simulink model "samerHARDWARE"  (R2025b)
settings: Solver=FixedStepDiscrete  StartTime=0.0  StopTime=1500  FixedStep=0.05  RelTol=1e-3
libraries: slpidlib x6
(part 1 of 2)
settings Model: SimulationMode=external  Creator=Ahmed Sedky  LastModifiedBy=Samer FARAJ
settings OptimizationCC: EnhancedBackFolding=on  PassReuseOutputArgsAs=Individual arguments  ZeroExternalMemoryAtStartup=off  ZeroInternalMemoryAtStartup=off  MaxStackSize=64  OptimizeBlockOrder=speed  DifferentSizesBufferReuse=on  OptimizationCustomize=off  EfficientTunableParamExpr=on
settings DebuggingCC: ParameterTunabilityLossMsg=error
settings HardwareCC: ProdBitPerInt=16.0  ProdBitPerPointer=16.0  ProdBitPerSizeT=16.0  ProdBitPerPtrDiffT=16.0  ProdLargestAtomicFloat=None  ProdWordSize=8.0  ProdHWDeviceType=Atmel->AVR
settings SFSimCC: MATLABDynamicMemAlloc=off
settings RTWCC: SystemTargetFile=ert.tlc  TLCOptions=-aExtModeXCPSimulationTimeInTicks=1 -aExtModeXCPClassicInterface=0  TemplateMakefile=ert_default_tmf  Toolchain=Arduino AVR  BuildConfiguration=Faster Runs  GPUComputeCapability=3.5  Description=Embedded Coder
settings CodeAppCC: ForceParamTrailComments=on  IgnoreCustomStorageClasses=off  OperatorAnnotations=on  SimulinkDataObjDesc=on  SFDataObjDesc=on  InsertBlockDesc=on
settings ERTTargetCC: ExtMode=on  ExtModeTransport=3.0  ExtModeStaticAlloc=on  ExtModeStaticAllocSize=2048.0  ExtModeMexFile=ext_xcp  ExtModeMexArgs=0 4 921600  ExtModeIntrfLevel=Level2 - Open  InlinedParameterPlacement=Hierarchical  ERTCustomFileTemplate=example_file_process.tlc  DynamicArrayContainerType=coder::array  SupportContinuousTime=on

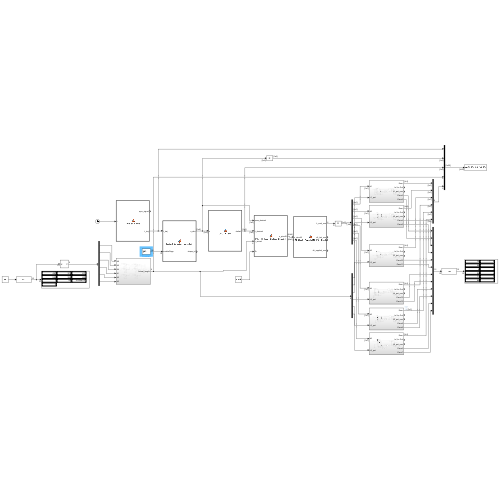
[thumbnail: Simulink's stored preview of the top-level diagram]
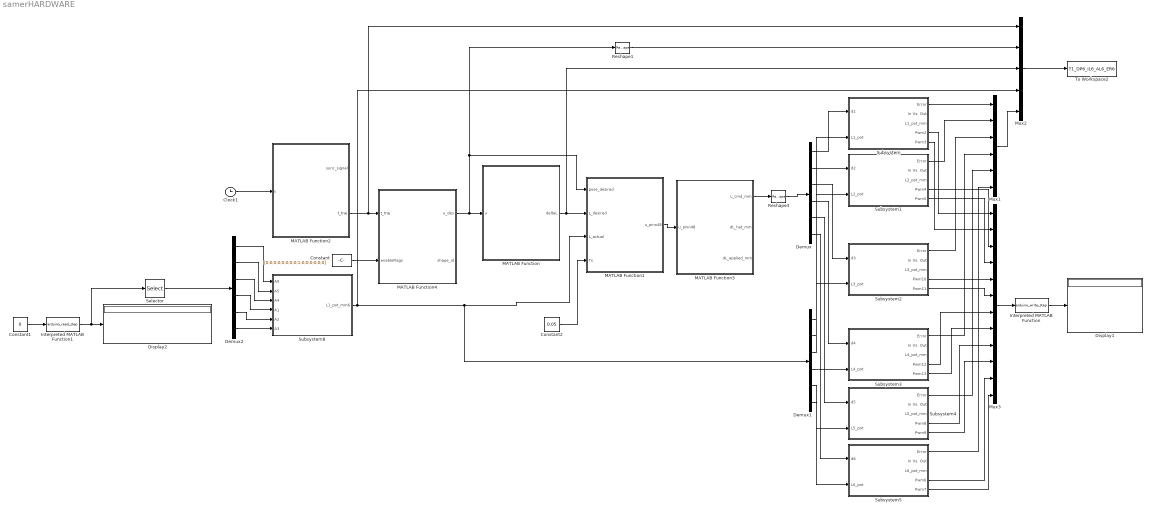
== system samerHARDWARE ==
  Clock1 : Clock
  Constant : Constant  Value=[0;0;0;0;0;0;0;0;1;0;0;0;0;0;0]
  Constant1 : Constant  Value=0
  Constant2 : Constant  Value=0.05
  Demux : Demux  Outputs=6
  Demux1 : Demux  Outputs=6
  Demux2 : Demux  Outputs=6
  Display1 : Display
  Display2 : Display
  Interpreted MATLAB Function : MATLABFcn  MATLABFcn=arduino_write_step  OutputDimensions=12  OutputSignalType=real
  Interpreted MATLAB Function1 : MATLABFcn  MATLABFcn=arduino_read_step  OutputDimensions=10  OutputSignalType=real
  MATLAB Function : MATLAB Function  TreatAsAtomicUnit=on
  MATLAB Function1 : MATLAB Function  TreatAsAtomicUnit=on
  MATLAB Function2 : MATLAB Function  TreatAsAtomicUnit=on
  MATLAB Function3 : MATLAB Function  TreatAsAtomicUnit=on
  MATLAB Function4 : MATLAB Function  TreatAsAtomicUnit=on
  Mux1 : Mux  Inputs=6
  Mux2 : Mux  Inputs=5
  Mux3 : Mux  Inputs=12
  Reshape1 : Reshape  OutputDimensionality=Customize  OutputDimensions=[1,6]
  Reshape3 : Reshape  OutputDimensionality=Customize  OutputDimensions=[1,6]
  Selector : Selector  InputPortWidth=10  IndexOptions=Index vector (dialog)  Indices=[1:6]  OutputSizes=1
  Subsystem : Subsystem
  Subsystem1 : Subsystem
  Subsystem2 : Subsystem
  Subsystem3 : Subsystem
  Subsystem4 : Subsystem
  Subsystem5 : Subsystem
  Subsystem8 : Subsystem
  To Workspace2 : ToWorkspace  VariableName=T1_DP6_IL6_AL6_ER6  SampleTime=-1
      settings: Save2DSignal=2-D array (concatenate along first dimension)
  wires:
  Constant1/1 -> Interpreted MATLAB Function1/1
  Interpreted MATLAB Function1/1 -> Selector/1, Display2/1
  Demux2/4 -> Subsystem8/4(A1)
  Demux2/3 -> Subsystem8/3(A4)
  Subsystem8/1(L1_pot_mm6) -> Demux1/1, MATLAB Function1/3(L_actual), Mux2/4
  Demux2/6 -> Subsystem8/6(A3)
  Demux2/2 -> Subsystem8/2(A5)
  Subsystem/5(Pwm3) -> Mux3/2
  Subsystem/1(Error) -> Mux1/1
  Selector/1 -> Demux2/1
  Demux1/5 -> Subsystem4/2(L5_pot)
  Demux1/1 -> Subsystem/2(L1_pot)
  Demux/5 -> Subsystem4/1(d5)
  Demux2/1 -> Subsystem8/1(A0)
  Clock1/1 -> MATLAB Function2/1(t)
  Interpreted MATLAB Function/1 -> Display1/1
  Demux2/5 -> Subsystem8/5(A2)
  Mux3/1 -> Interpreted MATLAB Function/1
  Subsystem1/1(Error) -> Mux1/2
  MATLAB Function2/2(t_traj) -> Mux2/1, MATLAB Function4/1(t_traj)
  Constant2/1 -> MATLAB Function1/4(Ts)
  Constant/1 -> MATLAB Function4/2(enableFlags)
  MATLAB Function4/1(u_des) -> Reshape1/1, MATLAB Function1/1(pose_desired), MATLAB Function/1(u)
  Subsystem1/5(Pwm5) -> Mux3/4
  Subsystem4/5(Pwm9) -> Mux3/10
  Subsystem3/4(Pwm12) -> Mux3/7
  MATLAB Function/1(deltaL) -> MATLAB Function1/2(L_desired), Mux2/3
  Reshape1/1 -> Mux2/2
  MATLAB Function1/1(u_pinn48) -> MATLAB Function3/1(u_pinn48)
  Subsystem5/1(Error) -> Mux1/6
  MATLAB Function3/1(L_cmd_mm) -> Reshape3/1
  Reshape3/1 -> Demux/1
  Demux/1 -> Subsystem/1(d1)
  Subsystem2/4(Pwm10) -> Mux3/5
  Demux1/6 -> Subsystem5/2(L6_pot)
  Demux1/2 -> Subsystem1/2(L2_pot)
  Demux/6 -> Subsystem5/1(d6)
  Demux/2 -> Subsystem1/1(d2)
  Demux1/3 -> Subsystem2/2(L3_pot)
  Demux/3 -> Subsystem2/1(d3)
  Demux1/4 -> Subsystem3/2(L4_pot)
  Demux/4 -> Subsystem3/1(d4)
  Subsystem/4(Pwm2) -> Mux3/1
  Subsystem5/4(Pwm6) -> Mux3/11
  Subsystem1/4(Pwm4) -> Mux3/3
  Subsystem2/1(Error) -> Mux1/3
  Subsystem2/5(Pwm11) -> Mux3/6
  Subsystem3/1(Error) -> Mux1/4
  Subsystem3/5(Pwm13) -> Mux3/8
  Subsystem4/1(Error) -> Mux1/5
  Subsystem4/4(Pwm8) -> Mux3/9
  Subsystem5/5(Pwm7) -> Mux3/12
  Mux2/1 -> To Workspace2/1
  Mux1/1 -> Mux2/5

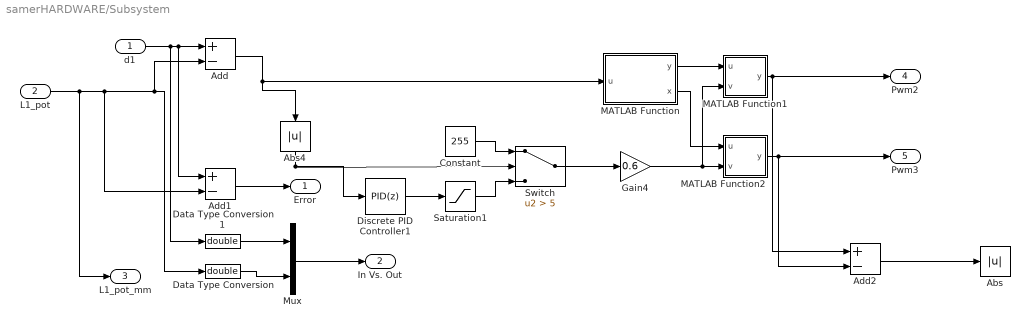
== system samerHARDWARE/Subsystem ==
  d1 : Inport
  L1_pot : Inport  Port=2
  Abs : Abs  SaturateOnIntegerOverflow=off
  Abs4 : Abs  SaturateOnIntegerOverflow=off
  Add : Sum  Inputs=+-
  Add1 : Sum  Inputs=+-
  Add2 : Sum  Inputs=+-
  Constant : Constant  Value=255
  Data Type Conversion : DataTypeConversion  OutDataTypeStr=double  SaturateOnIntegerOverflow=off  RndMeth=Floor
  Data Type Conversion1 : DataTypeConversion  OutDataTypeStr=double  SaturateOnIntegerOverflow=off  RndMeth=Floor
  Discrete PID Controller1 : slpidlib/PID Controller  Controller=PID  Form=Parallel  TimeDomain=Discrete-time  UseExternalTs=off  SampleTime=0.05  IntegratorMethod=Forward Euler  FilterMethod=Forward Euler  ControllerParametersSource=internal  P=175  I=0  UseKiTs=off  D=0.75  UseExternalDerivativeSource=off  N=1  UseFilter=on  TunerSelectOption=Transfer Function Based (PID Tuner App)  InitialConditionSource=internal  InitialConditionForIntegrator=0  InitialConditionForFilter=0  DifferentiatorICPrevScaledInput=0  ExternalReset=none  TrackingMode=off  Kt=1  LimitOutput=off  SatLimitsSource=internal  UpperSaturationLimit=inf  LowerSaturationLimit=-inf  LinearizeAsGain=off  AntiWindupMode=none  Kb=1  LimitIntegrator=off  UpperIntegratorSaturationLimit=inf  LowerIntegratorSaturationLimit=-inf  POutMin=[]  POutMax=[]  IOutMin=[]  IOutMax=[]  DOutMin=[]  DOutMax=[]  NOutMin=[]  NOutMax=[]  SumOutMin=[]  SumOutMax=[]  SaturationOutMin=[]  SaturationOutMax=[]  PParamMin=[]  PParamMax=[]  IParamMin=[]  IParamMax=[]  DParamMin=[]  DParamMax=[]  NParamMin=[]  NParamMax=[]  KbParamMin=[]  KbParamMax=[]  KtParamMin=[]  KtParamMax=[]  KbOutMin=[]  KbOutMax=[]  KtOutMin=[]  KtOutMax=[]  IntegratorOutMin=[]  IntegratorOutMax=[]  FilterOutMin=[]  FilterOutMax=[]  SumI1OutMin=[]  SumI1OutMax=[]  SumI2OutMin=[]  SumI2OutMax=[]  SumI3OutMin=[]  SumI3OutMax=[]  SumI4OutMin=[]  SumI4OutMax=[]  SumDOutMin=[]  SumDOutMax=[]  DifferentiatorOutMin=[]  DifferentiatorOutMax=[]  FilterDiffOutCoefMin=[]  FilterDiffOutCoefMax=[]  ReciprocalOutMin=[]  ReciprocalOutMax=[]  SumDenOutMin=[]  SumDenOutMax=[]  SumNumOutMin=[]  SumNumOutMax=[]  DivideOutMin=[]  DivideOutMax=[]  UdiffTsProdOutMin=[]  UdiffTsProdOutMax=[]  NTsProdOutMin=[]  NTsProdOutMax=[]  UintegralTsProdOutMin=[]  UintegralTsProdOutMax=[]  UngainTsProdOutMin=[]  UngainTsProdOutMax=[]  ClampingZeroOutDataTypeStr=Inherit: Inherit via back propagation  ClampingZeroOutMin=[]  ClampingZeroOutMax=[]  FilterDenConstantOutDataTypeStr=Inherit: Inherit via back propagation  FilterDenConstantOutMin=[]  FilterDenConstantOutMax=[]  PCopyOutDataTypeStr=Inherit: Inherit via back propagation  PCopyOutMin=[]  PCopyOutMax=[]  NCopyOutDataTypeStr=Inherit: Inherit via back propagation  NCopyOutMin=[]  NCopyOutMax=[]  IntegratorContinuousStateAttributes=''  IntegratorStateMustResolveToSignalObject=off  IntegratorRTWStateStorageClass=Auto  FilterContinuousStateAttributes=''  FilterStateMustResolveToSignalObject=off  FilterRTWStateStorageClass=Auto  ParallelPVariant=InternalParameters  IdealPVariant=Disabled  IVariant=InternalParameters  DVariant=InternalParameters  IntegratorVariant=Discrete  SatVariant=Disabled  AWVariant=Passthrough  PCopyVariant=Disabled  TRVariant=Disabled  FdbkBlocksVariant=Forward  IdealPFdbkVariant=Disabled  SatFdbkVariant=Disabled  DerivativeFilterVariant=ForwardEulerFilter  NVariant=InternalParameters  NCopyVariant=Disabled  FilterICVariant=InternalICsFilter  IntegratorICVariant=InternalICs  ExternalResetVariant=Disabled  TRSumVariant=Passthrough  SumFdbkVariant=Disabled  SumVariant=Sum_PID  TsampFilterVariant=InternalTs  TsampNgainVariant=Passthrough  TsampIntegralVariant=Disabled_SignalSpec  ExternalSaturationOutDataTypeStr=Inherit: Same as second input  DerivativeSourceVariant=ErrorSignal  PreIntVariant=InternalPreInt
      settings: LibrarySourceBlock=simulink/Discrete/Discrete PID Controller
  Gain4 : Gain  Gain=0.6
  MATLAB Function : MATLAB Function  TreatAsAtomicUnit=on
  MATLAB Function1 : MATLAB Function  TreatAsAtomicUnit=on
  MATLAB Function2 : MATLAB Function  TreatAsAtomicUnit=on
  Mux : Mux  Inputs=2
  Saturation1 : Saturate  UpperLimit=220  LowerLimit=0
  Switch : Switch  Criteria=u2 > Threshold  Threshold=5  SaturateOnIntegerOverflow=off  InputSameDT=off
  Error : Outport
  In Vs. Out : Outport  Port=2
  L1_pot_mm : Outport  Port=3
  Pwm2 : Outport  Port=4
  Pwm3 : Outport  Port=5
  wires:
  Data Type Conversion1/1 -> Mux/1
  d1/1 -> Add1/1, Add/1, Data Type Conversion1/1
  Abs4/1 -> Discrete PID Controller1/1, Switch/2
  Add1/1 -> Error/1
  Add/1 -> Abs4/1, MATLAB Function/1(u)
  Data Type Conversion/1 -> Mux/2
  Mux/1 -> In Vs. Out/1
  Discrete PID Controller1/1 -> Saturation1/1
  Add2/1 -> Abs/1
  Constant/1 -> Switch/1
  Saturation1/1 -> Switch/3
  Switch/1 -> Gain4/1
  MATLAB Function/1(y) -> MATLAB Function1/1(u)
  Gain4/1 -> MATLAB Function1/2(v), MATLAB Function2/2(v)
  MATLAB Function/2(x) -> MATLAB Function2/1(u)
  MATLAB Function2/1(y) -> Pwm3/1, Add2/2
  L1_pot/1 -> L1_pot_mm/1, Add1/2, Add/2, Data Type Conversion/1
  MATLAB Function1/1(y) -> Pwm2/1, Add2/1

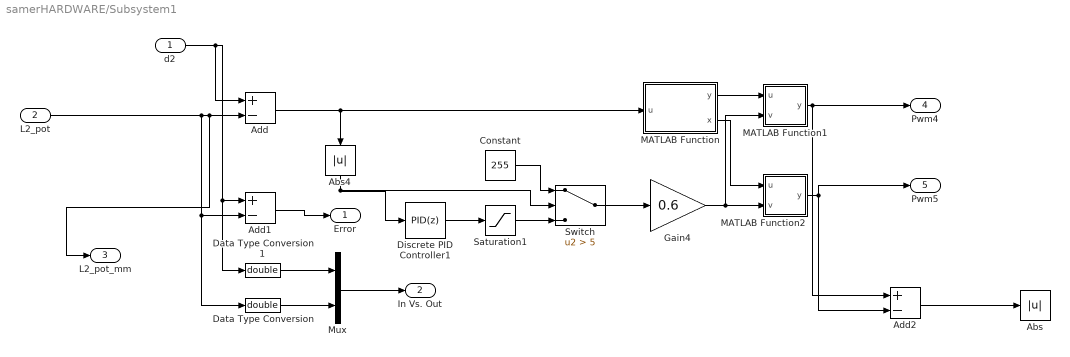
== system samerHARDWARE/Subsystem1 ==
  d2 : Inport
  L2_pot : Inport  Port=2
  Abs : Abs  SaturateOnIntegerOverflow=off
  Abs4 : Abs  SaturateOnIntegerOverflow=off
  Add : Sum  Inputs=+-
  Add1 : Sum  Inputs=+-
  Add2 : Sum  Inputs=+-
  Constant : Constant  Value=255
  Data Type Conversion : DataTypeConversion  OutDataTypeStr=double  SaturateOnIntegerOverflow=off  RndMeth=Floor
  Data Type Conversion1 : DataTypeConversion  OutDataTypeStr=double  SaturateOnIntegerOverflow=off  RndMeth=Floor
  Discrete PID Controller1 : slpidlib/PID Controller  Controller=PID  Form=Parallel  TimeDomain=Discrete-time  UseExternalTs=off  SampleTime=0.05  IntegratorMethod=Forward Euler  FilterMethod=Forward Euler  ControllerParametersSource=internal  P=175  I=0  UseKiTs=off  D=0.75  UseExternalDerivativeSource=off  N=1  UseFilter=off  TunerSelectOption=Transfer Function Based (PID Tuner App)  InitialConditionSource=internal  InitialConditionForIntegrator=0  InitialConditionForFilter=0  DifferentiatorICPrevScaledInput=0  ExternalReset=none  TrackingMode=off  Kt=1  LimitOutput=off  SatLimitsSource=internal  UpperSaturationLimit=inf  LowerSaturationLimit=-inf  LinearizeAsGain=off  AntiWindupMode=none  Kb=1  LimitIntegrator=off  UpperIntegratorSaturationLimit=inf  LowerIntegratorSaturationLimit=-inf  POutMin=[]  POutMax=[]  IOutMin=[]  IOutMax=[]  DOutMin=[]  DOutMax=[]  NOutMin=[]  NOutMax=[]  SumOutMin=[]  SumOutMax=[]  SaturationOutMin=[]  SaturationOutMax=[]  PParamMin=[]  PParamMax=[]  IParamMin=[]  IParamMax=[]  DParamMin=[]  DParamMax=[]  NParamMin=[]  NParamMax=[]  KbParamMin=[]  KbParamMax=[]  KtParamMin=[]  KtParamMax=[]  KbOutMin=[]  KbOutMax=[]  KtOutMin=[]  KtOutMax=[]  IntegratorOutMin=[]  IntegratorOutMax=[]  FilterOutMin=[]  FilterOutMax=[]  SumI1OutMin=[]  SumI1OutMax=[]  SumI2OutMin=[]  SumI2OutMax=[]  SumI3OutMin=[]  SumI3OutMax=[]  SumI4OutMin=[]  SumI4OutMax=[]  SumDOutMin=[]  SumDOutMax=[]  DifferentiatorOutMin=[]  DifferentiatorOutMax=[]  FilterDiffOutCoefMin=[]  FilterDiffOutCoefMax=[]  ReciprocalOutMin=[]  ReciprocalOutMax=[]  SumDenOutMin=[]  SumDenOutMax=[]  SumNumOutMin=[]  SumNumOutMax=[]  DivideOutMin=[]  DivideOutMax=[]  UdiffTsProdOutMin=[]  UdiffTsProdOutMax=[]  NTsProdOutMin=[]  NTsProdOutMax=[]  UintegralTsProdOutMin=[]  UintegralTsProdOutMax=[]  UngainTsProdOutMin=[]  UngainTsProdOutMax=[]  ClampingZeroOutDataTypeStr=Inherit: Inherit via back propagation  ClampingZeroOutMin=[]  ClampingZeroOutMax=[]  FilterDenConstantOutDataTypeStr=Inherit: Inherit via back propagation  FilterDenConstantOutMin=[]  FilterDenConstantOutMax=[]  PCopyOutDataTypeStr=Inherit: Inherit via back propagation  PCopyOutMin=[]  PCopyOutMax=[]  NCopyOutDataTypeStr=Inherit: Inherit via back propagation  NCopyOutMin=[]  NCopyOutMax=[]  IntegratorContinuousStateAttributes=''  IntegratorStateMustResolveToSignalObject=off  IntegratorRTWStateStorageClass=Auto  FilterContinuousStateAttributes=''  FilterStateMustResolveToSignalObject=off  FilterRTWStateStorageClass=Auto  ParallelPVariant=InternalParameters  IdealPVariant=Disabled  IVariant=InternalParameters  DVariant=InternalParameters  IntegratorVariant=Discrete  SatVariant=Disabled  AWVariant=Passthrough  PCopyVariant=Disabled  TRVariant=Disabled  FdbkBlocksVariant=Forward  IdealPFdbkVariant=Disabled  SatFdbkVariant=Disabled  DerivativeFilterVariant=Differentiator  NVariant=Passthrough  NCopyVariant=Disabled_SignalSpec  FilterICVariant=InternalICsDifferentiator  IntegratorICVariant=InternalICs  ExternalResetVariant=Disabled  TRSumVariant=Passthrough  SumFdbkVariant=Disabled  SumVariant=Sum_PID  TsampFilterVariant=InternalTs  TsampNgainVariant=Passthrough  TsampIntegralVariant=Disabled_SignalSpec  ExternalSaturationOutDataTypeStr=Inherit: Same as second input  DerivativeSourceVariant=ErrorSignal  PreIntVariant=InternalPreInt
      settings: LibrarySourceBlock=simulink/Discrete/Discrete PID Controller
  Gain4 : Gain  Gain=0.6
  MATLAB Function : MATLAB Function  TreatAsAtomicUnit=on
  MATLAB Function1 : MATLAB Function  TreatAsAtomicUnit=on
  MATLAB Function2 : MATLAB Function  TreatAsAtomicUnit=on
  Mux : Mux  Inputs=2
  Saturation1 : Saturate  UpperLimit=220  LowerLimit=0
  Switch : Switch  Criteria=u2 > Threshold  Threshold=5  SaturateOnIntegerOverflow=off  InputSameDT=off
  Error : Outport
  In Vs. Out : Outport  Port=2
  L2_pot_mm : Outport  Port=3
  Pwm4 : Outport  Port=4
  Pwm5 : Outport  Port=5
  wires:
  MATLAB Function/1(y) -> MATLAB Function1/1(u)
  d2/1 -> Data Type Conversion1/1, Add1/1, Add/1
  MATLAB Function/2(x) -> MATLAB Function2/1(u)
  L2_pot/1 -> Data Type Conversion/1, Add1/2, L2_pot_mm/1, Add/2
  Add2/1 -> Abs/1
  Add/1 -> Abs4/1, MATLAB Function/1(u)
  Constant/1 -> Switch/1
  Abs4/1 -> Discrete PID Controller1/1, Switch/2
  Add1/1 -> Error/1
  Gain4/1 -> MATLAB Function2/2(v), MATLAB Function1/2(v)
  Data Type Conversion1/1 -> Mux/1
  Data Type Conversion/1 -> Mux/2
  Mux/1 -> In Vs. Out/1
  Discrete PID Controller1/1 -> Saturation1/1
  Saturation1/1 -> Switch/3
  Switch/1 -> Gain4/1
  MATLAB Function2/1(y) -> Pwm5/1, Add2/2
  MATLAB Function1/1(y) -> Pwm4/1, Add2/1

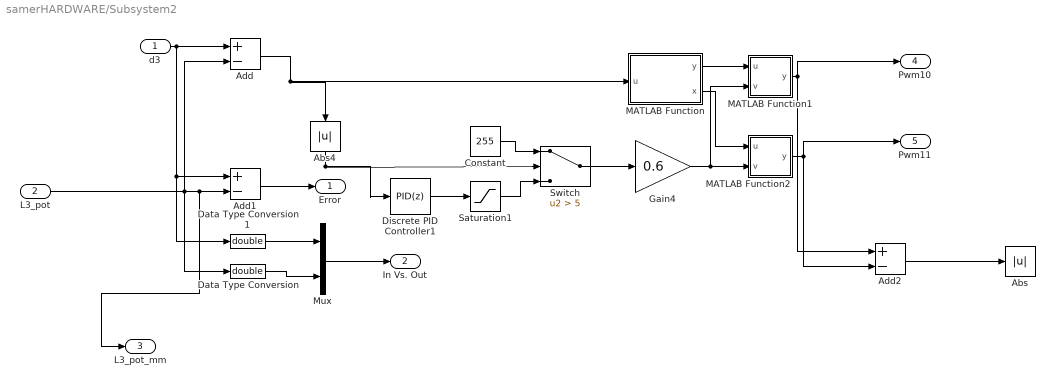
== system samerHARDWARE/Subsystem2 ==
  d3 : Inport
  L3_pot : Inport  Port=2
  Abs : Abs  SaturateOnIntegerOverflow=off
  Abs4 : Abs  SaturateOnIntegerOverflow=off
  Add : Sum  Inputs=+-
  Add1 : Sum  Inputs=+-
  Add2 : Sum  Inputs=+-
  Constant : Constant  Value=255
  Data Type Conversion : DataTypeConversion  OutDataTypeStr=double  SaturateOnIntegerOverflow=off  RndMeth=Floor
  Data Type Conversion1 : DataTypeConversion  OutDataTypeStr=double  SaturateOnIntegerOverflow=off  RndMeth=Floor
  Discrete PID Controller1 : slpidlib/PID Controller  Controller=PID  Form=Parallel  TimeDomain=Discrete-time  UseExternalTs=off  SampleTime=0.05  IntegratorMethod=Forward Euler  FilterMethod=Forward Euler  ControllerParametersSource=internal  P=175  I=0  UseKiTs=off  D=0.75  UseExternalDerivativeSource=off  N=1  UseFilter=off  TunerSelectOption=Transfer Function Based (PID Tuner App)  InitialConditionSource=internal  InitialConditionForIntegrator=0  InitialConditionForFilter=0  DifferentiatorICPrevScaledInput=0  ExternalReset=none  TrackingMode=off  Kt=1  LimitOutput=off  SatLimitsSource=internal  UpperSaturationLimit=inf  LowerSaturationLimit=-inf  LinearizeAsGain=off  AntiWindupMode=none  Kb=1  LimitIntegrator=off  UpperIntegratorSaturationLimit=inf  LowerIntegratorSaturationLimit=-inf  POutMin=[]  POutMax=[]  IOutMin=[]  IOutMax=[]  DOutMin=[]  DOutMax=[]  NOutMin=[]  NOutMax=[]  SumOutMin=[]  SumOutMax=[]  SaturationOutMin=[]  SaturationOutMax=[]  PParamMin=[]  PParamMax=[]  IParamMin=[]  IParamMax=[]  DParamMin=[]  DParamMax=[]  NParamMin=[]  NParamMax=[]  KbParamMin=[]  KbParamMax=[]  KtParamMin=[]  KtParamMax=[]  KbOutMin=[]  KbOutMax=[]  KtOutMin=[]  KtOutMax=[]  IntegratorOutMin=[]  IntegratorOutMax=[]  FilterOutMin=[]  FilterOutMax=[]  SumI1OutMin=[]  SumI1OutMax=[]  SumI2OutMin=[]  SumI2OutMax=[]  SumI3OutMin=[]  SumI3OutMax=[]  SumI4OutMin=[]  SumI4OutMax=[]  SumDOutMin=[]  SumDOutMax=[]  DifferentiatorOutMin=[]  DifferentiatorOutMax=[]  FilterDiffOutCoefMin=[]  FilterDiffOutCoefMax=[]  ReciprocalOutMin=[]  ReciprocalOutMax=[]  SumDenOutMin=[]  SumDenOutMax=[]  SumNumOutMin=[]  SumNumOutMax=[]  DivideOutMin=[]  DivideOutMax=[]  UdiffTsProdOutMin=[]  UdiffTsProdOutMax=[]  NTsProdOutMin=[]  NTsProdOutMax=[]  UintegralTsProdOutMin=[]  UintegralTsProdOutMax=[]  UngainTsProdOutMin=[]  UngainTsProdOutMax=[]  ClampingZeroOutDataTypeStr=Inherit: Inherit via back propagation  ClampingZeroOutMin=[]  ClampingZeroOutMax=[]  FilterDenConstantOutDataTypeStr=Inherit: Inherit via back propagation  FilterDenConstantOutMin=[]  FilterDenConstantOutMax=[]  PCopyOutDataTypeStr=Inherit: Inherit via back propagation  PCopyOutMin=[]  PCopyOutMax=[]  NCopyOutDataTypeStr=Inherit: Inherit via back propagation  NCopyOutMin=[]  NCopyOutMax=[]  IntegratorContinuousStateAttributes=''  IntegratorStateMustResolveToSignalObject=off  IntegratorRTWStateStorageClass=Auto  FilterContinuousStateAttributes=''  FilterStateMustResolveToSignalObject=off  FilterRTWStateStorageClass=Auto  ParallelPVariant=InternalParameters  IdealPVariant=Disabled  IVariant=InternalParameters  DVariant=InternalParameters  IntegratorVariant=Discrete  SatVariant=Disabled  AWVariant=Passthrough  PCopyVariant=Disabled  TRVariant=Disabled  FdbkBlocksVariant=Forward  IdealPFdbkVariant=Disabled  SatFdbkVariant=Disabled  DerivativeFilterVariant=Differentiator  NVariant=Passthrough  NCopyVariant=Disabled_SignalSpec  FilterICVariant=InternalICsDifferentiator  IntegratorICVariant=InternalICs  ExternalResetVariant=Disabled  TRSumVariant=Passthrough  SumFdbkVariant=Disabled  SumVariant=Sum_PID  TsampFilterVariant=InternalTs  TsampNgainVariant=Passthrough  TsampIntegralVariant=Disabled_SignalSpec  ExternalSaturationOutDataTypeStr=Inherit: Same as second input  DerivativeSourceVariant=ErrorSignal  PreIntVariant=InternalPreInt
      settings: LibrarySourceBlock=simulink/Discrete/Discrete PID Controller
  Gain4 : Gain  Gain=0.6
  MATLAB Function : MATLAB Function  TreatAsAtomicUnit=on
  MATLAB Function1 : MATLAB Function  TreatAsAtomicUnit=on
  MATLAB Function2 : MATLAB Function  TreatAsAtomicUnit=on
  Mux : Mux  Inputs=2
  Saturation1 : Saturate  UpperLimit=220  LowerLimit=0
  Switch : Switch  Criteria=u2 > Threshold  Threshold=5  SaturateOnIntegerOverflow=off  InputSameDT=off
  Error : Outport
  In Vs. Out : Outport  Port=2
  L3_pot_mm : Outport  Port=3
  Pwm10 : Outport  Port=4
  Pwm11 : Outport  Port=5
  wires:
  Abs4/1 -> Discrete PID Controller1/1, Switch/2
  Add1/1 -> Error/1
  d3/1 -> Data Type Conversion1/1, Add1/1, Add/1
  Data Type Conversion/1 -> Mux/2
  Constant/1 -> Switch/1
  L3_pot/1 -> Data Type Conversion/1, L3_pot_mm/1, Add1/2, Add/2
  Add2/1 -> Abs/1
  Add/1 -> Abs4/1, MATLAB Function/1(u)
  Gain4/1 -> MATLAB Function2/2(v), MATLAB Function1/2(v)
  Data Type Conversion1/1 -> Mux/1
  Mux/1 -> In Vs. Out/1
  Discrete PID Controller1/1 -> Saturation1/1
  Saturation1/1 -> Switch/3
  Switch/1 -> Gain4/1
  MATLAB Function/1(y) -> MATLAB Function1/1(u)
  MATLAB Function/2(x) -> MATLAB Function2/1(u)
  MATLAB Function1/1(y) -> Pwm10/1, Add2/1
  MATLAB Function2/1(y) -> Pwm11/1, Add2/2

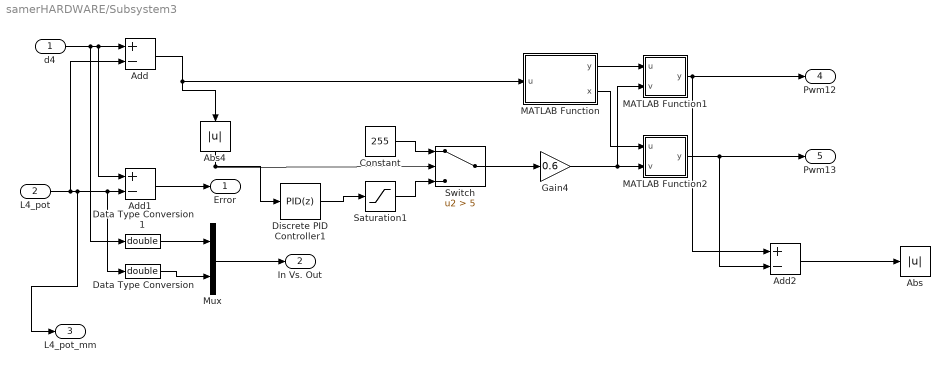
== system samerHARDWARE/Subsystem3 ==
  d4 : Inport
  L4_pot : Inport  Port=2
  Abs : Abs  SaturateOnIntegerOverflow=off
  Abs4 : Abs  SaturateOnIntegerOverflow=off
  Add : Sum  Inputs=+-
  Add1 : Sum  Inputs=+-
  Add2 : Sum  Inputs=+-
  Constant : Constant  Value=255
  Data Type Conversion : DataTypeConversion  OutDataTypeStr=double  SaturateOnIntegerOverflow=off  RndMeth=Floor
  Data Type Conversion1 : DataTypeConversion  OutDataTypeStr=double  SaturateOnIntegerOverflow=off  RndMeth=Floor
  Discrete PID Controller1 : slpidlib/PID Controller  Controller=PID  Form=Parallel  TimeDomain=Discrete-time  UseExternalTs=off  SampleTime=0.05  IntegratorMethod=Forward Euler  FilterMethod=Forward Euler  ControllerParametersSource=internal  P=175  I=0  UseKiTs=off  D=0.75  UseExternalDerivativeSource=off  N=1  UseFilter=off  TunerSelectOption=Transfer Function Based (PID Tuner App)  InitialConditionSource=internal  InitialConditionForIntegrator=0  InitialConditionForFilter=0  DifferentiatorICPrevScaledInput=0  ExternalReset=none  TrackingMode=off  Kt=1  LimitOutput=off  SatLimitsSource=internal  UpperSaturationLimit=inf  LowerSaturationLimit=-inf  LinearizeAsGain=off  AntiWindupMode=none  Kb=1  LimitIntegrator=off  UpperIntegratorSaturationLimit=inf  LowerIntegratorSaturationLimit=-inf  POutMin=[]  POutMax=[]  IOutMin=[]  IOutMax=[]  DOutMin=[]  DOutMax=[]  NOutMin=[]  NOutMax=[]  SumOutMin=[]  SumOutMax=[]  SaturationOutMin=[]  SaturationOutMax=[]  PParamMin=[]  PParamMax=[]  IParamMin=[]  IParamMax=[]  DParamMin=[]  DParamMax=[]  NParamMin=[]  NParamMax=[]  KbParamMin=[]  KbParamMax=[]  KtParamMin=[]  KtParamMax=[]  KbOutMin=[]  KbOutMax=[]  KtOutMin=[]  KtOutMax=[]  IntegratorOutMin=[]  IntegratorOutMax=[]  FilterOutMin=[]  FilterOutMax=[]  SumI1OutMin=[]  SumI1OutMax=[]  SumI2OutMin=[]  SumI2OutMax=[]  SumI3OutMin=[]  SumI3OutMax=[]  SumI4OutMin=[]  SumI4OutMax=[]  SumDOutMin=[]  SumDOutMax=[]  DifferentiatorOutMin=[]  DifferentiatorOutMax=[]  FilterDiffOutCoefMin=[]  FilterDiffOutCoefMax=[]  ReciprocalOutMin=[]  ReciprocalOutMax=[]  SumDenOutMin=[]  SumDenOutMax=[]  SumNumOutMin=[]  SumNumOutMax=[]  DivideOutMin=[]  DivideOutMax=[]  UdiffTsProdOutMin=[]  UdiffTsProdOutMax=[]  NTsProdOutMin=[]  NTsProdOutMax=[]  UintegralTsProdOutMin=[]  UintegralTsProdOutMax=[]  UngainTsProdOutMin=[]  UngainTsProdOutMax=[]  ClampingZeroOutDataTypeStr=Inherit: Inherit via back propagation  ClampingZeroOutMin=[]  ClampingZeroOutMax=[]  FilterDenConstantOutDataTypeStr=Inherit: Inherit via back propagation  FilterDenConstantOutMin=[]  FilterDenConstantOutMax=[]  PCopyOutDataTypeStr=Inherit: Inherit via back propagation  PCopyOutMin=[]  PCopyOutMax=[]  NCopyOutDataTypeStr=Inherit: Inherit via back propagation  NCopyOutMin=[]  NCopyOutMax=[]  IntegratorContinuousStateAttributes=''  IntegratorStateMustResolveToSignalObject=off  IntegratorRTWStateStorageClass=Auto  FilterContinuousStateAttributes=''  FilterStateMustResolveToSignalObject=off  FilterRTWStateStorageClass=Auto  ParallelPVariant=InternalParameters  IdealPVariant=Disabled  IVariant=InternalParameters  DVariant=InternalParameters  IntegratorVariant=Discrete  SatVariant=Disabled  AWVariant=Passthrough  PCopyVariant=Disabled  TRVariant=Disabled  FdbkBlocksVariant=Forward  IdealPFdbkVariant=Disabled  SatFdbkVariant=Disabled  DerivativeFilterVariant=Differentiator  NVariant=Passthrough  NCopyVariant=Disabled_SignalSpec  FilterICVariant=InternalICsDifferentiator  IntegratorICVariant=InternalICs  ExternalResetVariant=Disabled  TRSumVariant=Passthrough  SumFdbkVariant=Disabled  SumVariant=Sum_PID  TsampFilterVariant=InternalTs  TsampNgainVariant=Passthrough  TsampIntegralVariant=Disabled_SignalSpec  ExternalSaturationOutDataTypeStr=Inherit: Same as second input  DerivativeSourceVariant=ErrorSignal  PreIntVariant=InternalPreInt
      settings: LibrarySourceBlock=simulink/Discrete/Discrete PID Controller
  Gain4 : Gain  Gain=0.6
  MATLAB Function : MATLAB Function  TreatAsAtomicUnit=on
  MATLAB Function1 : MATLAB Function  TreatAsAtomicUnit=on
  MATLAB Function2 : MATLAB Function  TreatAsAtomicUnit=on
  Mux : Mux  Inputs=2
  Saturation1 : Saturate  UpperLimit=220  LowerLimit=0
  Switch : Switch  Criteria=u2 > Threshold  Threshold=5  SaturateOnIntegerOverflow=off  InputSameDT=off
  Error : Outport
  In Vs. Out : Outport  Port=2
  L4_pot_mm : Outport  Port=3
  Pwm12 : Outport  Port=4
  Pwm13 : Outport  Port=5
  wires:
  Add2/1 -> Abs/1
  Gain4/1 -> MATLAB Function2/2(v), MATLAB Function1/2(v)
  d4/1 -> Add1/1, Add/1, Data Type Conversion1/1
  MATLAB Function/2(x) -> MATLAB Function2/1(u)
  L4_pot/1 -> L4_pot_mm/1, Data Type Conversion/1, Add1/2, Add/2
  Add/1 -> Abs4/1, MATLAB Function/1(u)
  Add1/1 -> Error/1
  Data Type Conversion1/1 -> Mux/1
  Data Type Conversion/1 -> Mux/2
  Abs4/1 -> Discrete PID Controller1/1, Switch/2
  Mux/1 -> In Vs. Out/1
  Discrete PID Controller1/1 -> Saturation1/1
  Constant/1 -> Switch/1
  MATLAB Function2/1(y) -> Pwm13/1, Add2/2
  Saturation1/1 -> Switch/3
  Switch/1 -> Gain4/1
  MATLAB Function/1(y) -> MATLAB Function1/1(u)
  MATLAB Function1/1(y) -> Pwm12/1, Add2/1

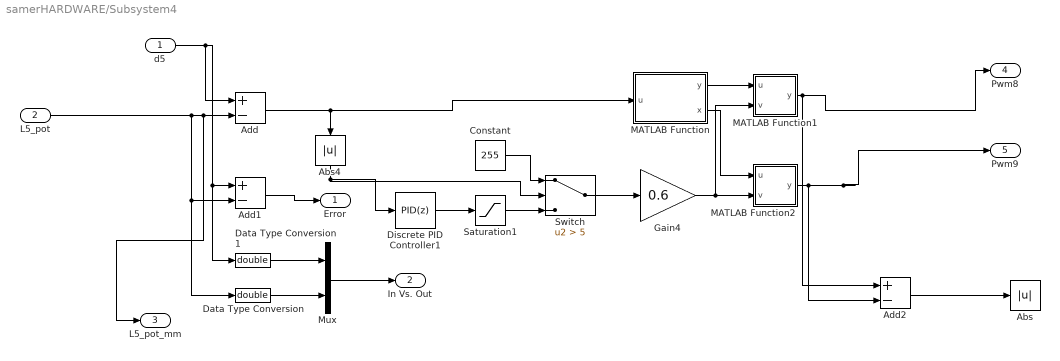
== system samerHARDWARE/Subsystem4 ==
  d5 : Inport
  L5_pot : Inport  Port=2
  Abs : Abs  SaturateOnIntegerOverflow=off
  Abs4 : Abs  SaturateOnIntegerOverflow=off
  Add : Sum  Inputs=+-
  Add1 : Sum  Inputs=+-
  Add2 : Sum  Inputs=+-
  Constant : Constant  Value=255
  Data Type Conversion : DataTypeConversion  OutDataTypeStr=double  SaturateOnIntegerOverflow=off  RndMeth=Floor
  Data Type Conversion1 : DataTypeConversion  OutDataTypeStr=double  SaturateOnIntegerOverflow=off  RndMeth=Floor
  Discrete PID Controller1 : slpidlib/PID Controller  Controller=PID  Form=Parallel  TimeDomain=Discrete-time  UseExternalTs=off  SampleTime=0.05  IntegratorMethod=Forward Euler  FilterMethod=Forward Euler  ControllerParametersSource=internal  P=175  I=0  UseKiTs=off  D=0.75  UseExternalDerivativeSource=off  N=1  UseFilter=off  TunerSelectOption=Transfer Function Based (PID Tuner App)  InitialConditionSource=internal  InitialConditionForIntegrator=0  InitialConditionForFilter=0  DifferentiatorICPrevScaledInput=0  ExternalReset=none  TrackingMode=off  Kt=1  LimitOutput=off  SatLimitsSource=internal  UpperSaturationLimit=inf  LowerSaturationLimit=-inf  LinearizeAsGain=off  AntiWindupMode=none  Kb=1  LimitIntegrator=off  UpperIntegratorSaturationLimit=inf  LowerIntegratorSaturationLimit=-inf  POutMin=[]  POutMax=[]  IOutMin=[]  IOutMax=[]  DOutMin=[]  DOutMax=[]  NOutMin=[]  NOutMax=[]  SumOutMin=[]  SumOutMax=[]  SaturationOutMin=[]  SaturationOutMax=[]  PParamMin=[]  PParamMax=[]  IParamMin=[]  IParamMax=[]  DParamMin=[]  DParamMax=[]  NParamMin=[]  NParamMax=[]  KbParamMin=[]  KbParamMax=[]  KtParamMin=[]  KtParamMax=[]  KbOutMin=[]  KbOutMax=[]  KtOutMin=[]  KtOutMax=[]  IntegratorOutMin=[]  IntegratorOutMax=[]  FilterOutMin=[]  FilterOutMax=[]  SumI1OutMin=[]  SumI1OutMax=[]  SumI2OutMin=[]  SumI2OutMax=[]  SumI3OutMin=[]  SumI3OutMax=[]  SumI4OutMin=[]  SumI4OutMax=[]  SumDOutMin=[]  SumDOutMax=[]  DifferentiatorOutMin=[]  DifferentiatorOutMax=[]  FilterDiffOutCoefMin=[]  FilterDiffOutCoefMax=[]  ReciprocalOutMin=[]  ReciprocalOutMax=[]  SumDenOutMin=[]  SumDenOutMax=[]  SumNumOutMin=[]  SumNumOutMax=[]  DivideOutMin=[]  DivideOutMax=[]  UdiffTsProdOutMin=[]  UdiffTsProdOutMax=[]  NTsProdOutMin=[]  NTsProdOutMax=[]  UintegralTsProdOutMin=[]  UintegralTsProdOutMax=[]  UngainTsProdOutMin=[]  UngainTsProdOutMax=[]  ClampingZeroOutDataTypeStr=Inherit: Inherit via back propagation  ClampingZeroOutMin=[]  ClampingZeroOutMax=[]  FilterDenConstantOutDataTypeStr=Inherit: Inherit via back propagation  FilterDenConstantOutMin=[]  FilterDenConstantOutMax=[]  PCopyOutDataTypeStr=Inherit: Inherit via back propagation  PCopyOutMin=[]  PCopyOutMax=[]  NCopyOutDataTypeStr=Inherit: Inherit via back propagation  NCopyOutMin=[]  NCopyOutMax=[]  IntegratorContinuousStateAttributes=''  IntegratorStateMustResolveToSignalObject=off  IntegratorRTWStateStorageClass=Auto  FilterContinuousStateAttributes=''  FilterStateMustResolveToSignalObject=off  FilterRTWStateStorageClass=Auto  ParallelPVariant=InternalParameters  IdealPVariant=Disabled  IVariant=InternalParameters  DVariant=InternalParameters  IntegratorVariant=Discrete  SatVariant=Disabled  AWVariant=Passthrough  PCopyVariant=Disabled  TRVariant=Disabled  FdbkBlocksVariant=Forward  IdealPFdbkVariant=Disabled  SatFdbkVariant=Disabled  DerivativeFilterVariant=Differentiator  NVariant=Passthrough  NCopyVariant=Disabled_SignalSpec  FilterICVariant=InternalICsDifferentiator  IntegratorICVariant=InternalICs  ExternalResetVariant=Disabled  TRSumVariant=Passthrough  SumFdbkVariant=Disabled  SumVariant=Sum_PID  TsampFilterVariant=InternalTs  TsampNgainVariant=Passthrough  TsampIntegralVariant=Disabled_SignalSpec  ExternalSaturationOutDataTypeStr=Inherit: Same as second input  DerivativeSourceVariant=ErrorSignal  PreIntVariant=InternalPreInt
      settings: LibrarySourceBlock=simulink/Discrete/Discrete PID Controller
  Gain4 : Gain  Gain=0.6
  MATLAB Function : MATLAB Function  TreatAsAtomicUnit=on
  MATLAB Function1 : MATLAB Function  TreatAsAtomicUnit=on
  MATLAB Function2 : MATLAB Function  TreatAsAtomicUnit=on
  Mux : Mux  Inputs=2
  Saturation1 : Saturate  UpperLimit=220  LowerLimit=0
  Switch : Switch  Criteria=u2 > Threshold  Threshold=5  SaturateOnIntegerOverflow=off  InputSameDT=off
  Error : Outport
  In Vs. Out : Outport  Port=2
  L5_pot_mm : Outport  Port=3
  Pwm8 : Outport  Port=4
  Pwm9 : Outport  Port=5
  wires:
  Add2/1 -> Abs/1
  MATLAB Function1/1(y) -> Pwm8/1, Add2/1
  d5/1 -> Data Type Conversion1/1, Add1/1, Add/1
  L5_pot/1 -> Data Type Conversion/1, Add1/2, L5_pot_mm/1, Add/2
  Add/1 -> Abs4/1, MATLAB Function/1(u)
  Add1/1 -> Error/1
  Data Type Conversion1/1 -> Mux/1
  Data Type Conversion/1 -> Mux/2
  Constant/1 -> Switch/1
  Abs4/1 -> Switch/2, Discrete PID Controller1/1
  Mux/1 -> In Vs. Out/1
  Discrete PID Controller1/1 -> Saturation1/1
  Saturation1/1 -> Switch/3
  Switch/1 -> Gain4/1
  MATLAB Function/1(y) -> MATLAB Function1/1(u)
  MATLAB Function/2(x) -> MATLAB Function2/1(u)
  Gain4/1 -> MATLAB Function2/2(v), MATLAB Function1/2(v)
  MATLAB Function2/1(y) -> Add2/2, Pwm9/1

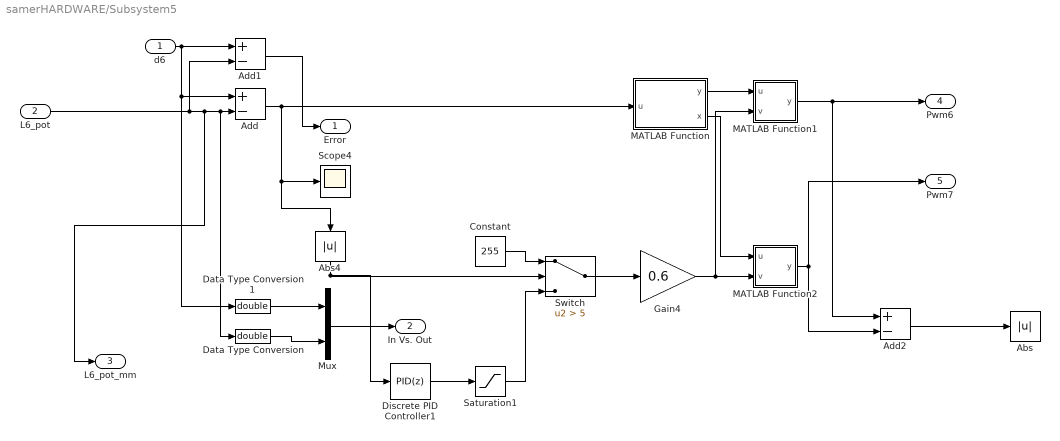
== system samerHARDWARE/Subsystem5 ==
  d6 : Inport
  L6_pot : Inport  Port=2
  Abs : Abs  SaturateOnIntegerOverflow=off
  Abs4 : Abs  SaturateOnIntegerOverflow=off
  Add : Sum  Inputs=+-
  Add1 : Sum  Inputs=+-
  Add2 : Sum  Inputs=+-
  Constant : Constant  Value=255
  Data Type Conversion : DataTypeConversion  OutDataTypeStr=double  SaturateOnIntegerOverflow=off  RndMeth=Floor
  Data Type Conversion1 : DataTypeConversion  OutDataTypeStr=double  SaturateOnIntegerOverflow=off  RndMeth=Floor
  Discrete PID Controller1 : slpidlib/PID Controller  Controller=PID  Form=Parallel  TimeDomain=Discrete-time  UseExternalTs=off  SampleTime=0.05  IntegratorMethod=Forward Euler  FilterMethod=Forward Euler  ControllerParametersSource=internal  P=175  I=0  UseKiTs=off  D=0.75  UseExternalDerivativeSource=off  N=1  UseFilter=off  TunerSelectOption=Transfer Function Based (PID Tuner App)  InitialConditionSource=internal  InitialConditionForIntegrator=0  InitialConditionForFilter=0  DifferentiatorICPrevScaledInput=0  ExternalReset=none  TrackingMode=off  Kt=1  LimitOutput=off  SatLimitsSource=internal  UpperSaturationLimit=inf  LowerSaturationLimit=-inf  LinearizeAsGain=off  AntiWindupMode=none  Kb=1  LimitIntegrator=off  UpperIntegratorSaturationLimit=inf  LowerIntegratorSaturationLimit=-inf  POutMin=[]  POutMax=[]  IOutMin=[]  IOutMax=[]  DOutMin=[]  DOutMax=[]  NOutMin=[]  NOutMax=[]  SumOutMin=[]  SumOutMax=[]  SaturationOutMin=[]  SaturationOutMax=[]  PParamMin=[]  PParamMax=[]  IParamMin=[]  IParamMax=[]  DParamMin=[]  DParamMax=[]  NParamMin=[]  NParamMax=[]  KbParamMin=[]  KbParamMax=[]  KtParamMin=[]  KtParamMax=[]  KbOutMin=[]  KbOutMax=[]  KtOutMin=[]  KtOutMax=[]  IntegratorOutMin=[]  IntegratorOutMax=[]  FilterOutMin=[]  FilterOutMax=[]  SumI1OutMin=[]  SumI1OutMax=[]  SumI2OutMin=[]  SumI2OutMax=[]  SumI3OutMin=[]  SumI3OutMax=[]  SumI4OutMin=[]  SumI4OutMax=[]  SumDOutMin=[]  SumDOutMax=[]  DifferentiatorOutMin=[]  DifferentiatorOutMax=[]  FilterDiffOutCoefMin=[]  FilterDiffOutCoefMax=[]  ReciprocalOutMin=[]  ReciprocalOutMax=[]  SumDenOutMin=[]  SumDenOutMax=[]  SumNumOutMin=[]  SumNumOutMax=[]  DivideOutMin=[]  DivideOutMax=[]  UdiffTsProdOutMin=[]  UdiffTsProdOutMax=[]  NTsProdOutMin=[]  NTsProdOutMax=[]  UintegralTsProdOutMin=[]  UintegralTsProdOutMax=[]  UngainTsProdOutMin=[]  UngainTsProdOutMax=[]  ClampingZeroOutDataTypeStr=Inherit: Inherit via back propagation  ClampingZeroOutMin=[]  ClampingZeroOutMax=[]  FilterDenConstantOutDataTypeStr=Inherit: Inherit via back propagation  FilterDenConstantOutMin=[]  FilterDenConstantOutMax=[]  PCopyOutDataTypeStr=Inherit: Inherit via back propagation  PCopyOutMin=[]  PCopyOutMax=[]  NCopyOutDataTypeStr=Inherit: Inherit via back propagation  NCopyOutMin=[]  NCopyOutMax=[]  IntegratorContinuousStateAttributes=''  IntegratorStateMustResolveToSignalObject=off  IntegratorRTWStateStorageClass=Auto  FilterContinuousStateAttributes=''  FilterStateMustResolveToSignalObject=off  FilterRTWStateStorageClass=Auto  ParallelPVariant=InternalParameters  IdealPVariant=Disabled  IVariant=InternalParameters  DVariant=InternalParameters  IntegratorVariant=Discrete  SatVariant=Disabled  AWVariant=Passthrough  PCopyVariant=Disabled  TRVariant=Disabled  FdbkBlocksVariant=Forward  IdealPFdbkVariant=Disabled  SatFdbkVariant=Disabled  DerivativeFilterVariant=Differentiator  NVariant=Passthrough  NCopyVariant=Disabled_SignalSpec  FilterICVariant=InternalICsDifferentiator  IntegratorICVariant=InternalICs  ExternalResetVariant=Disabled  TRSumVariant=Passthrough  SumFdbkVariant=Disabled  SumVariant=Sum_PID  TsampFilterVariant=InternalTs  TsampNgainVariant=Passthrough  TsampIntegralVariant=Disabled_SignalSpec  ExternalSaturationOutDataTypeStr=Inherit: Same as second input  DerivativeSourceVariant=ErrorSignal  PreIntVariant=InternalPreInt
      settings: LibrarySourceBlock=simulink/Discrete/Discrete PID Controller
  Gain4 : Gain  Gain=0.6
  MATLAB Function : MATLAB Function  TreatAsAtomicUnit=on
  MATLAB Function1 : MATLAB Function  TreatAsAtomicUnit=on
  MATLAB Function2 : MATLAB Function  TreatAsAtomicUnit=on
  Mux : Mux  Inputs=2
  Saturation1 : Saturate  UpperLimit=220  LowerLimit=0
  Scope4 : Scope
      settings: ActiveDisplayYMinimum=-38.33565  ActiveDisplayYMaximum=48.7182
  Switch : Switch  Criteria=u2 > Threshold  Threshold=5  SaturateOnIntegerOverflow=off  InputSameDT=off
  Error : Outport
  In Vs. Out : Outport  Port=2
  L6_pot_mm : Outport  Port=3
  Pwm6 : Outport  Port=4
  Pwm7 : Outport  Port=5
  wires:
  Add1/1 -> Error/1
  Add2/1 -> Abs/1
  Gain4/1 -> MATLAB Function2/2(v), MATLAB Function1/2(v)
  d6/1 -> Data Type Conversion1/1, Add/1, Add1/1
  MATLAB Function/2(x) -> MATLAB Function2/1(u)
  L6_pot/1 -> L6_pot_mm/1, Data Type Conversion/1, Add/2, Add1/2
  Add/1 -> Scope4/1, Abs4/1, MATLAB Function/1(u)
  Data Type Conversion1/1 -> Mux/1
  Data Type Conversion/1 -> Mux/2
  Constant/1 -> Switch/1
  Abs4/1 -> Discrete PID Controller1/1, Switch/2
  Mux/1 -> In Vs. Out/1
  Discrete PID Controller1/1 -> Saturation1/1
  Saturation1/1 -> Switch/3
  Switch/1 -> Gain4/1
  MATLAB Function/1(y) -> MATLAB Function1/1(u)
  MATLAB Function1/1(y) -> Pwm6/1, Add2/1
  MATLAB Function2/1(y) -> Pwm7/1, Add2/2

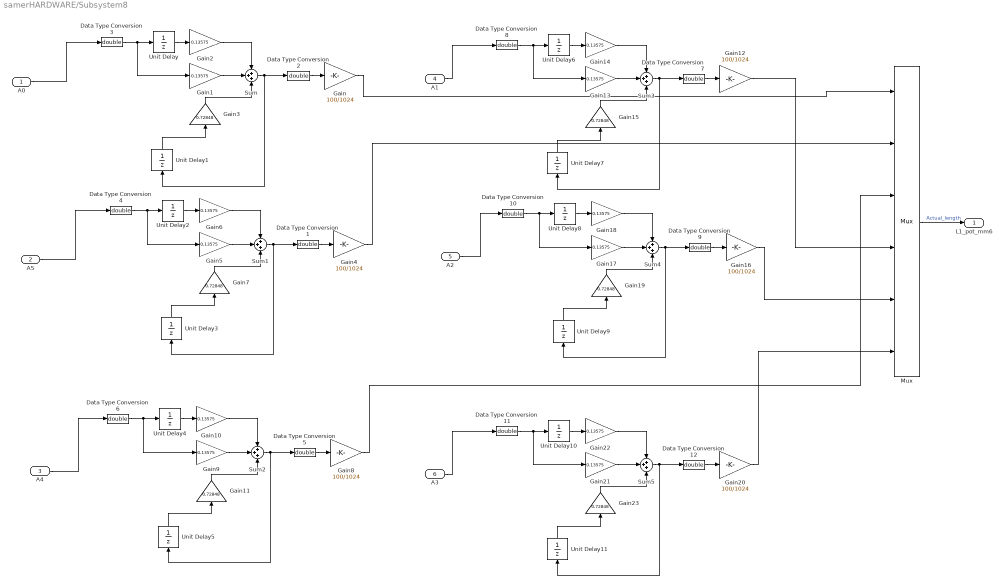
== system samerHARDWARE/Subsystem8 ==
  A0 : Inport
  A5 : Inport  Port=2
  A4 : Inport  Port=3
  A1 : Inport  Port=4
  A2 : Inport  Port=5
  A3 : Inport  Port=6
  Data Type Conversion{1..12} (12 alike) : DataTypeConversion  OutDataTypeStr=double  SaturateOnIntegerOverflow=off  RndMeth=Floor
  Gain{,4,8,12,16,20} (6 alike) : Gain  Gain=100/1024
  Gain{1..2,5..6,9..10,13..14,17..18,21..22} (12 alike) : Gain  Gain=0.13575
  Gain{3,7,11,15,19,23} (6 alike) : Gain  Gain=0.72848
  Mux : Mux  Inputs=6
  Sum{,1..5} (6 alike) : Sum  Inputs=+++
  Unit Delay{,1..11} (12 alike) : UnitDelay  SampleTime=-1  HasFrameUpgradeWarning=on
  L1_pot_mm6 : Outport
  wires:
  A0/1 -> Data Type Conversion3/1
  Data Type Conversion2/1 -> Gain/1
  Gain1/1 -> Sum/2
  Data Type Conversion3/1 -> Gain1/1, Unit Delay/1
  Gain2/1 -> Sum/1
  Unit Delay1/1 -> Gain3/1
  Unit Delay/1 -> Gain2/1
  Gain3/1 -> Sum/3
  Sum/1 -> Data Type Conversion2/1, Unit Delay1/1
  Gain/1 -> Mux/1
  Gain4/1 -> Mux/2
  Data Type Conversion4/1 -> Gain5/1, Unit Delay2/1
  Data Type Conversion1/1 -> Gain4/1
  Gain6/1 -> Sum1/1
  Gain7/1 -> Sum1/3
  Unit Delay2/1 -> Gain6/1
  Gain5/1 -> Sum1/2
  Sum1/1 -> Data Type Conversion1/1, Unit Delay3/1
  Unit Delay3/1 -> Gain7/1
  A5/1 -> Data Type Conversion4/1
  Gain8/1 -> Mux/3
  Data Type Conversion6/1 -> Gain9/1, Unit Delay4/1
  Data Type Conversion5/1 -> Gain8/1
  Gain10/1 -> Sum2/1
  Gain11/1 -> Sum2/3
  Unit Delay4/1 -> Gain10/1
  Gain9/1 -> Sum2/2
  Sum2/1 -> Data Type Conversion5/1, Unit Delay5/1
  Unit Delay5/1 -> Gain11/1
  A4/1 -> Data Type Conversion6/1
  Gain12/1 -> Mux/4
  Data Type Conversion8/1 -> Gain13/1, Unit Delay6/1
  Data Type Conversion7/1 -> Gain12/1
  Gain14/1 -> Sum3/1
  Gain15/1 -> Sum3/3
  Unit Delay6/1 -> Gain14/1
  Gain13/1 -> Sum3/2
  Sum3/1 -> Data Type Conversion7/1, Unit Delay7/1
  Unit Delay7/1 -> Gain15/1
  A1/1 -> Data Type Conversion8/1
  Gain16/1 -> Mux/5
  Data Type Conversion10/1 -> Gain17/1, Unit Delay8/1
  Data Type Conversion9/1 -> Gain16/1
  Gain18/1 -> Sum4/1
  Gain19/1 -> Sum4/3
  Unit Delay8/1 -> Gain18/1
  Gain17/1 -> Sum4/2
  Sum4/1 -> Data Type Conversion9/1, Unit Delay9/1
  Unit Delay9/1 -> Gain19/1
  A3/1 -> Data Type Conversion11/1
  Unit Delay11/1 -> Gain23/1
  Unit Delay10/1 -> Gain22/1
  Gain21/1 -> Sum5/2
  Gain22/1 -> Sum5/1
  Gain23/1 -> Sum5/3
  Data Type Conversion11/1 -> Gain21/1, Unit Delay10/1
  Sum5/1 -> Data Type Conversion12/1, Unit Delay11/1
  Gain20/1 -> Mux/6
  Data Type Conversion12/1 -> Gain20/1
  Mux/1 -> L1_pot_mm6/1  "Actual_length"
  A2/1 -> Data Type Conversion10/1

== matlab function samerHARDWARE/Subsystem3/MATLAB Function ==
  data: u input; y output; x output
function [y,x] = fcn(u)

if u >= 0
    y=1;
    x=0;
else
    y=0;
    x=1;
end

== matlab function samerHARDWARE/Subsystem3/MATLAB Function1 ==
  data: u input; y output; v input
function y = fcn(u,v)

y = u*v;

== matlab function samerHARDWARE/Subsystem3/MATLAB Function2 ==
  data: u input; y output; v input
function y = fcn(u,v)

y = u*v;

== matlab function samerHARDWARE/Subsystem4/MATLAB Function ==
  data: u input; y output; x output
function [y,x] = fcn(u)

if u >= 0
    y=1;
    x=0;
else
    y=0;
    x=1;
end

== matlab function samerHARDWARE/Subsystem4/MATLAB Function1 ==
  data: u input; y output; v input
function y = fcn(u,v)

y = u*v;

== matlab function samerHARDWARE/Subsystem4/MATLAB Function2 ==
  data: u input; y output; v input
function y = fcn(u,v)

y = u*v;

== matlab function samerHARDWARE/Subsystem5/MATLAB Function ==
  data: u input; y output; x output
function [y,x] = fcn(u)

if u >= 0
    y=1;
    x=0;
else
    y=0;
    x=1;
end

== matlab function samerHARDWARE/Subsystem5/MATLAB Function1 ==
  data: u input; y output; v input
function y = fcn(u,v)

y = u*v;

== matlab function samerHARDWARE/Subsystem5/MATLAB Function2 ==
  data: u input; y output; v input
function y = fcn(u,v)

y = u*v;

== matlab function samerHARDWARE/MATLAB Function1 ==
  data: pose_desired input; u_pinn48 output; L_desired input; L_actual input; Ts input
function u_pinn48 = PINN48_Input_Builder_Simulink(pose_desired, L_desired, L_actual, Ts)
%#codegen
% Builds runtime-safe 48-input vector for powerful PC PINN.

persistent L_desired_prev L_actual_prev L_actual_prev2 initialized

if isempty(initialized)
    L_desired_prev = double(reshape(L_desired, [6,1]));
    L_actual_prev  = double(reshape(L_actual,  [6,1]));
    L_actual_prev2 = double(reshape(L_actual,  [6,1]));
    initialized = true;
end

pose_desired = double(reshape(pose_desired, [6,1]));
L_desired    = double(reshape(L_desired,    [6,1]));
L_actual     = double(reshape(L_actual,     [6,1]));

if Ts <= 0
    Ts = 0.05;
end

% Desired velocity at current step
vL_desired = (L_desired - L_desired_prev) ./ Ts;

% Desired direction
dirL_desired = zeros(6,1);
eps_vel = 0.5;

for i = 1:6
    if vL_desired(i) > eps_vel
        dirL_desired(i) = 1;
    elseif vL_desired(i) < -eps_vel
        dirL_desired(i) = -1;
    else
        dirL_desired(i) = 0;
    end
end

% Runtime-safe previous actual velocity
vL_actual_prev = (L_actual_prev - L_actual_prev2) ./ Ts;

% Runtime-safe previous actual direction
dirL_actual_prev = zeros(6,1);

for i = 1:6
    if vL_actual_prev(i) > eps_vel
        dirL_actual_prev(i) = 1;
    elseif vL_actual_prev(i) < -eps_vel
        dirL_actual_prev(i) = -1;
    else
        dirL_actual_prev(i) = 0;
    end
end

% Previous tracking error
error_prev = L_desired_prev - L_actual_prev;

% Build 48x1 input
u_pinn48 = [
    pose_desired
    L_desired
    L_actual_prev
    vL_desired
    dirL_desired
    vL_actual_prev
    dirL_actual_prev
    error_prev
];

% Update memory after building input
L_desired_prev = L_desired;
L_actual_prev2 = L_actual_prev;
L_actual_prev  = L_actual;

u_pinn48 = double(reshape(u_pinn48, [48,1]));
end

== matlab function samerHARDWARE/MATLAB Function2 ==
  data: t input; sync_signal output; t_traj output
function [sync_signal, t_traj] = sync_and_time(t)
%#codegen

% LED synchronization signal
if t < 2
    sync_signal = 1;
elseif t < 4
    sync_signal = 0;
elseif t <  10
    sync_signal = 1;
else
    sync_signal = 0;
end

% Delay trajectory start until after sync pattern
if t < 100
    t_traj = 0;
else
    t_traj = t - 100;
end
end

== matlab function samerHARDWARE/MATLAB Function3 ==
  data: u_pinn48 input; L_cmd_mm output; dL_hat_mm output; dL_applied_mm output
function [L_cmd_mm, dL_hat_mm, dL_applied_mm] = PINN_Block_Powerful48_PC_Simulink(u_pinn48)
%#codegen
% PC-side powerful 48-input Stewart PINN wrapper.
%
% u_pinn48 order:
%   1:6    pose_desired(k)
%   7:12   L_desired(k)
%   13:18  L_actual(k-1)
%   19:24  vL_desired(k)
%   25:30  dirL_desired(k)
%   31:36  vL_actual(k-1)
%   37:42  dirL_actual(k-1)
%   43:48  error(k-1)

coder.extrinsic('stewart_powerful48_predict_pc');

% =========================
% Safety settings
% =========================
alpha = 0.6;                % first test pure IK
correctionLimit_mm = 0.0;  % safe first correction clamp
predictionLimit_mm = 5.0;   % raw PINN prediction clamp

u = double(reshape(u_pinn48, [48,1]));

L_desired_mm = u(7:12);

% Predefine output size for Simulink
dL_hat_mm = zeros(6,1);

% Call trained PC model
dL_hat_mm = stewart_powerful48_predict_pc(u);
dL_hat_mm = double(reshape(dL_hat_mm, [6,1]));

% Clamp raw model output
dL_hat_mm = min(max(dL_hat_mm, -predictionLimit_mm), predictionLimit_mm);

% Apply correction gain and safety clamp
dL_applied_mm = alpha .* dL_hat_mm;
dL_applied_mm = min(max(dL_applied_mm, -correctionLimit_mm), correctionLimit_mm);

% Final actuator command
% IMPORTANT: use + because target was L_desired - L_actual
L_cmd_mm = L_desired_mm + dL_applied_mm;

L_cmd_mm      = double(reshape(L_cmd_mm, [6,1]));
dL_hat_mm     = double(reshape(dL_hat_mm, [6,1]));
dL_applied_mm = double(reshape(dL_applied_mm, [6,1]));
end
